simulink model "Expt1_19EE3FP28_Rushali_PartA"  (R2017a)
settings: Solver=VariableStepAuto  StartTime=0.0  StopTime=0.001  MaxStep=1e-4  RelTol=1e-3
libraries: powerlib x16
settings Model: Creator=Rushali  LastModifiedBy=Rushali

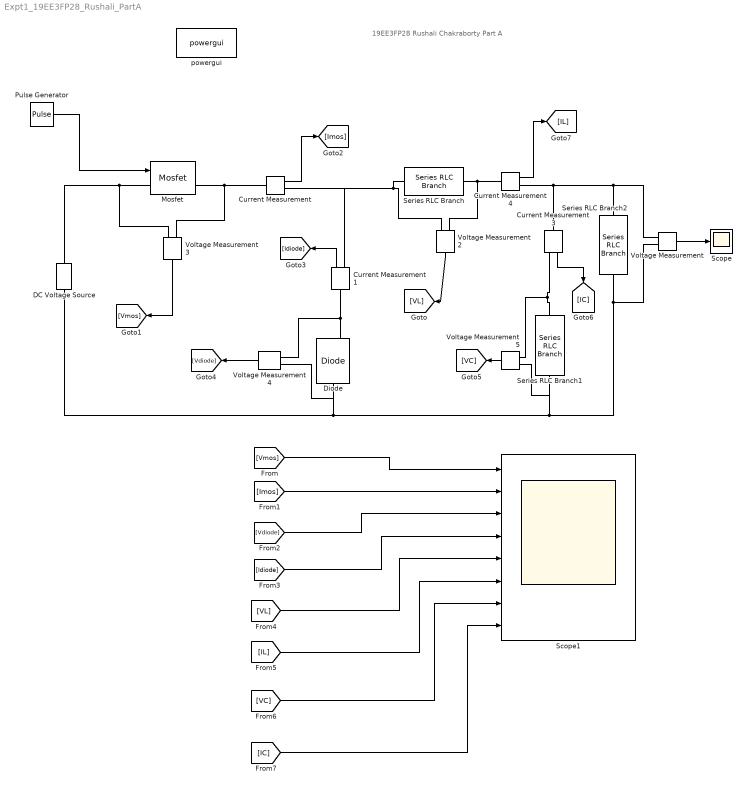
== system Expt1_19EE3FP28_Rushali_PartA ==
  note: 19EE3FP28
      | Rushali Chakraborty
      | Part A
  Current Measurement{,1,3..4} (4 alike) : powerlib/Measurements/Current Measurement  PhasorSimulation=off  OutputType=Complex  PSBequivalent=0
  DC Voltage Source : powerlib/Electrical Sources/DC Voltage Source  Amplitude=110  Measurements=None
  Diode : powerlib/Power Electronics/Diode  Ron=1e-6  Lon=0  Vf=0  IC=0  UseSnubber=0  Rs=500  Cs=250e-9  Measurements=on
  Mosfet : powerlib/Power Electronics/Mosfet  Ron=1e-6  Lon=0  Rd=1e-6  Vfd=0  IC=0  Rs=1e5  Cs=inf  Measurements=on
  Pulse Generator : DiscretePulseGenerator  PulseType=Time based  Period=1/50000  PulseWidth=50
  Scope : Scope
  Scope1 : Scope  NumInputPorts=8
  Series RLC Branch : powerlib/Elements/Series RLC Branch  LConnTagsString=__new0  RConnTagsString=__new0  BranchType=L  Resistance=1  Inductance=10e-6  SetiL0=off  InitialCurrent=0  Capacitance=1e-6  Setx0=off  InitialVoltage=0  Measurements=None
  Series RLC Branch1 : powerlib/Elements/Series RLC Branch  LConnTagsString=__new0  RConnTagsString=__new0  BranchType=C  Resistance=1  Inductance=1e-3  SetiL0=off  InitialCurrent=0  Capacitance=4e-6  Setx0=off  InitialVoltage=0  Measurements=None
  Series RLC Branch2 : powerlib/Elements/Series RLC Branch  LConnTagsString=__new0  RConnTagsString=__new0  BranchType=R  Resistance=11.52  Inductance=1e-3  SetiL0=off  InitialCurrent=0  Capacitance=1e-6  Setx0=off  InitialVoltage=0  Measurements=None
  Voltage Measurement{,2..5} (5 alike) : powerlib/Measurements/Voltage Measurement  PhasorSimulation=off  OutputType=Complex  PSBequivalent=0
  powergui : powerlib/powergui  Priority=1  SimulationMode=Continuous  SampleTime=50e-6  frequency=60  Iterations=50  frequencyindice=0  Pbase=100e6  ErrMax=1e-4  UnitsV=kV  UnitsW=MW  buscounter=0  FunctionMessages=off  echomessages=off  EnableUseOfTLC=off  CurrentSourceSwitches=off  DisableSnubberDevices=off  DisableRonSwitches=off  DisableVfSwitches=off  DisplayEquations=off  SolverType=Tustin/Backward Euler (TBE)  Interpol=off  ExternalGateDelay=off  methode=off  Ts=100  x0status=blocks  SPID=on  SwTol=0  HookPort=off  RestoreLinks=warning  ResistiveCurrentMeasurement=off  Frange=[0:2:500]  Ylog=off  Xlog=on  ShowGrid=off  save=off  variable=ZData  structure=0  ZoomFFT=off  StartTime=0.0  cycles=1  DisplayStyle=1  fundamental=60  FreqAxis=off  MaxFrequency=1000  frequencyindicesteady=1  RmsSteady=1  display=off
  wires:
  Pulse Generator/1 -> Mosfet/1
  Voltage Measurement/1 -> Scope/1
  Voltage Measurement2/1 -> [VL]
  Voltage Measurement3/1 -> [Vmos]
  Current Measurement/1 -> [Imos]
  Current Measurement1/1 -> [Idiode]
  Voltage Measurement4/1 -> [Vdiode]
  [Vmos] -> Scope1/1
  [Imos] -> Scope1/2
  [Vdiode] -> Scope1/3
  [Idiode] -> Scope1/4
  [VL] -> Scope1/5
  Voltage Measurement5/1 -> [VC]
  Current Measurement3/1 -> [IC]
  Current Measurement4/1 -> [IL]
  [IL] -> Scope1/6
  [VC] -> Scope1/7
  [IC] -> Scope1/8
  connections:
  Voltage Measurement2/LConn2 -- Series RLC Branch/RConn1 -- Current Measurement4/LConn1
  Voltage Measurement2/LConn1 -- Current Measurement1/RConn1 -- Current Measurement/RConn1 -- Series RLC Branch/LConn1
  Series RLC Branch2/RConn1 -- Voltage Measurement/LConn2 -- Voltage Measurement4/LConn1 -- Diode/LConn1 -- DC Voltage Source/LConn1 -- Voltage Measurement5/LConn2 -- Series RLC Branch1/RConn1
  DC Voltage Source/RConn1 -- Voltage Measurement3/LConn1 -- Mosfet/LConn1
  Mosfet/RConn1 -- Current Measurement/LConn1 -- Voltage Measurement3/LConn2
  Current Measurement1/LConn1 -- Voltage Measurement4/LConn2 -- Diode/RConn1
  Series RLC Branch1/LConn1 -- Voltage Measurement5/LConn1 -- Current Measurement3/RConn1
  Voltage Measurement/LConn1 -- Current Measurement4/RConn1 -- Current Measurement3/LConn1 -- Series RLC Branch2/LConn1
